simulink model "d3_model_MutiRateAndFractional"  (R2020a)
settings: Solver=VariableStepAuto  StartTime=0.0  StopTime=5e-2  RelTol=1e-3
libraries: dspsigops x6, simulink x2, dspfdesign x1, dspsrcs4 x1
settings Model: Creator=Marat  LastModifiedBy=Marat

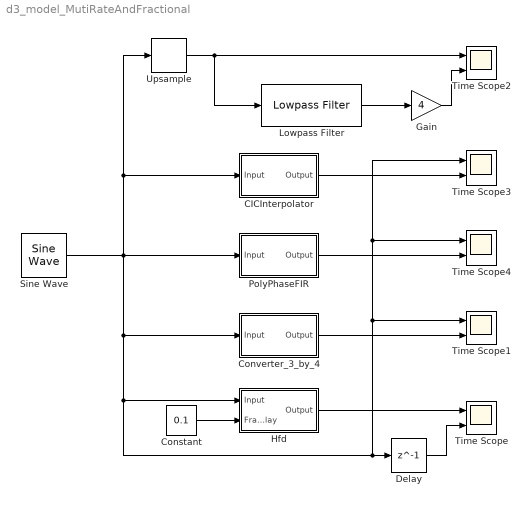
== system d3_model_MutiRateAndFractional ==
  CICInterpolator : Subsystem  Tag=FilterWizardSubSystem
      settings: ErrorFcn=dspFilterRealizedInBasicElemsAlgLoopErrFcnCallback
  Constant : Constant  Value=0.1
  Converter_3_by_4 : Subsystem  Tag=FilterWizardSubSystem
      settings: ErrorFcn=dspFilterRealizedInBasicElemsAlgLoopErrFcnCallback
  Delay : Delay  DelayLength=1
  Gain : Gain  Gain=4
  Hfd : Subsystem  Tag=FilterWizardSubSystem
      settings: ErrorFcn=dspFilterRealizedInBasicElemsAlgLoopErrFcnCallback
  Lowpass Filter : dspfdesign/Lowpass Filter  FilterType=FIR  DesignForMinimumOrder=on  FilterOrder=50  PassbandFrequency=100  StopbandFrequency=500  PassbandRipple=0.1  StopbandAttenuation=40  InheritSampleRate=on  SampleRate=44100  SimulateUsing=Interpreted execution  roundingMode=Floor  coeffsDataTypeStr=fixdt(1,16)
  PolyPhaseFIR : Subsystem  Tag=FilterWizardSubSystem
      settings: ErrorFcn=dspFilterRealizedInBasicElemsAlgLoopErrFcnCallback
  Sine Wave : dspsrcs4/Sine Wave  Amplitude=1  Frequency=50  Phase=0  SampleMode=Discrete  OutComplex=Real  CompMethod=Trigonometric fcn  TableSize=Speed  SampleTime=1/1000  SamplesPerFrame=1  ResetState=Restart at time zero  OutputFrames=off  dataType=double  wordLen=16  udDataType=sfix(16)  fracBitsMode=Best precision  numFracBits=15  OutDataTypeStr=double  LastOutDataTypeStr=double
  Time Scope{,1..4} (5 alike) : Scope  NumInputPorts=2
  Upsample : dspsigops/Upsample  N=4  phase=0  RateOptions=Allow multirate processing  ic=0  mode=Unused parameter value
  wires:
  Sine Wave/1 -> CICInterpolator/1(Input), Upsample/1, Converter_3_by_4/1(Input), Time Scope3/1, Time Scope4/1, Time Scope1/1, Delay/1, Hfd/1(Input), PolyPhaseFIR/1(Input)
  Constant/1 -> Hfd/2(FracDelay)
  Delay/1 -> Time Scope/2
  Converter_3_by_4/1(Output) -> Time Scope1/2
  Upsample/1 -> Time Scope2/1, Lowpass Filter/1
  Gain/1 -> Time Scope2/2
  Lowpass Filter/1 -> Gain/1
  CICInterpolator/1(Output) -> Time Scope3/2
  PolyPhaseFIR/1(Output) -> Time Scope4/2
  Hfd/1(Output) -> Time Scope/1

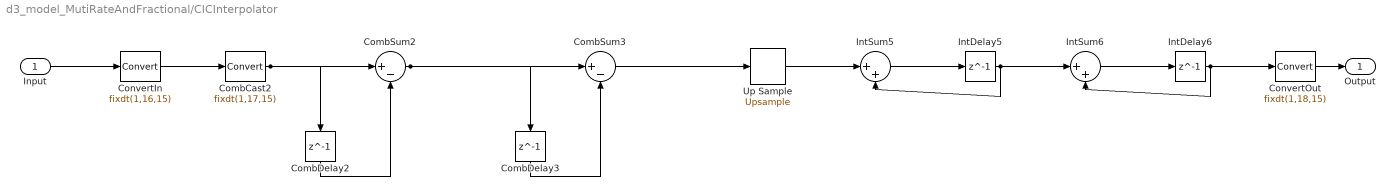
== system d3_model_MutiRateAndFractional/CICInterpolator ==
  Input : Inport
  CombCast2 : DataTypeConversion  OutDataTypeStr=fixdt(1,17,15)
  CombDelay2 : Delay  DelayLength=1  InitialCondition=0
  CombDelay3 : Delay  DelayLength=1  InitialCondition=0
  CombSum2 : Sum  Inputs=|+-  AccumDataTypeStr=fixdt(1,17,15)  OutDataTypeStr=fixdt(1,17,15)
  CombSum3 : Sum  Inputs=|+-  AccumDataTypeStr=fixdt(1,17,15)  OutDataTypeStr=fixdt(1,17,15)
  ConvertIn : DataTypeConversion  OutDataTypeStr=fixdt(1,16,15)  RndMeth=Nearest  SaturateOnIntegerOverflow=on
  ConvertOut : DataTypeConversion  OutDataTypeStr=fixdt(1,18,15)
  IntDelay5 : Delay  DelayLength=1  InitialCondition=0
  IntDelay6 : Delay  DelayLength=1  InitialCondition=0
  IntSum5 : Sum  Inputs=|++  AccumDataTypeStr=fixdt(1,17,15)  OutDataTypeStr=fixdt(1,17,15)
  IntSum6 : Sum  Inputs=|++  AccumDataTypeStr=fixdt(1,18,15)  OutDataTypeStr=fixdt(1,18,15)
  Up Sample : dspsigops/Upsample  N=4  phase=0  RateOptions=Allow multirate processing  ic=0  mode=Unused parameter value
  Output : Outport
  wires:
  Input/1 -> ConvertIn/1
  ConvertIn/1 -> CombCast2/1
  CombSum2/1 -> CombSum3/1, CombDelay3/1
  CombDelay2/1 -> CombSum2/2
  CombCast2/1 -> CombSum2/1, CombDelay2/1
  CombSum3/1 -> Up Sample/1
  CombDelay3/1 -> CombSum3/2
  Up Sample/1 -> IntSum5/1
  IntSum5/1 -> IntDelay5/1
  IntDelay5/1 -> IntSum5/2, IntSum6/1
  IntSum6/1 -> IntDelay6/1
  IntDelay6/1 -> IntSum6/2, ConvertOut/1
  ConvertOut/1 -> Output/1

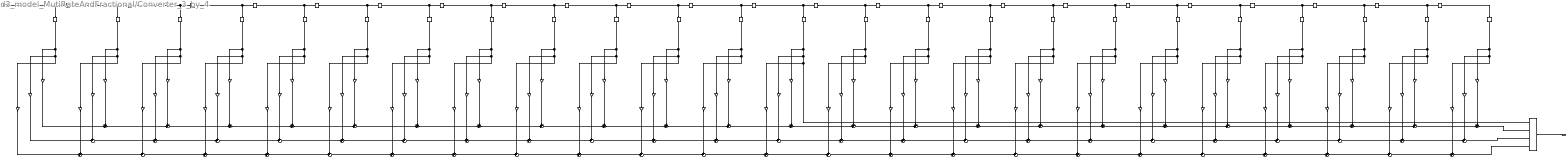
== system d3_model_MutiRateAndFractional/Converter_3_by_4 ==
  Input : Inport
  Delay{2..24} (23 alike) : Delay  DelayLength=1  InitialCondition=0
  FirsrcSys : Subsystem  Tag=FilterWizardSampleRateConverterCommutator
  RT{1..24} (24 alike) : RateTransition  Integrity=off  Deterministic=off  OutPortSampleTimeOpt=Multiple of input port sample time  OutPortSampleTimeMultiple=3/4
  p2(1) : Gain  Gain=-8.94209312709779976e-05  ParamDataTypeStr=double  RndMeth=Nearest  SaturateOnIntegerOverflow=on  OutDataTypeStr=Inherit: Same as input
  p2(10) : Gain  Gain=0.0673410868786561423  ParamDataTypeStr=double  RndMeth=Nearest  SaturateOnIntegerOverflow=on  OutDataTypeStr=Inherit: Same as input
  p2(11) : Gain  Gain=-0.118916504347217039  ParamDataTypeStr=double  RndMeth=Nearest  SaturateOnIntegerOverflow=on  OutDataTypeStr=Inherit: Same as input
  p2(12) : Gain  Gain=0.295831354115615619  ParamDataTypeStr=double  RndMeth=Nearest  SaturateOnIntegerOverflow=on  OutDataTypeStr=Inherit: Same as input
  p2(13) : Gain  Gain=0.898883674956074352  ParamDataTypeStr=double  RndMeth=Nearest  SaturateOnIntegerOverflow=on  OutDataTypeStr=Inherit: Same as input
  p2(14) : Gain  Gain=-0.173018480143057568  ParamDataTypeStr=double  RndMeth=Nearest  SaturateOnIntegerOverflow=on  OutDataTypeStr=Inherit: Same as input
  p2(15) : Gain  Gain=0.0878360099387300586  ParamDataTypeStr=double  RndMeth=Nearest  SaturateOnIntegerOverflow=on  OutDataTypeStr=Inherit: Same as input
  p2(16) : Gain  Gain=-0.0526648923165617677  ParamDataTypeStr=double  RndMeth=Nearest  SaturateOnIntegerOverflow=on  OutDataTypeStr=Inherit: Same as input
  p2(17) : Gain  Gain=0.0329540171313132749  ParamDataTypeStr=double  RndMeth=Nearest  SaturateOnIntegerOverflow=on  OutDataTypeStr=Inherit: Same as input
  p2(18) : Gain  Gain=-0.0205257309215202757  ParamDataTypeStr=double  RndMeth=Nearest  SaturateOnIntegerOverflow=on  OutDataTypeStr=Inherit: Same as input
  p2(19) : Gain  Gain=0.0123854962623023424  ParamDataTypeStr=double  RndMeth=Nearest  SaturateOnIntegerOverflow=on  OutDataTypeStr=Inherit: Same as input
  p2(2) : Gain  Gain=0.000410249281937617467  ParamDataTypeStr=double  RndMeth=Nearest  SaturateOnIntegerOverflow=on  OutDataTypeStr=Inherit: Same as input
  p2(20) : Gain  Gain=-0.00708453163123141071  ParamDataTypeStr=double  RndMeth=Nearest  SaturateOnIntegerOverflow=on  OutDataTypeStr=Inherit: Same as input
  p2(21) : Gain  Gain=0.00375215348431699822  ParamDataTypeStr=double  RndMeth=Nearest  SaturateOnIntegerOverflow=on  OutDataTypeStr=Inherit: Same as input
  p2(22) : Gain  Gain=-0.00178070447416222395  ParamDataTypeStr=double  RndMeth=Nearest  SaturateOnIntegerOverflow=on  OutDataTypeStr=Inherit: Same as input
  p2(23) : Gain  Gain=0.000714756913744617065  ParamDataTypeStr=double  RndMeth=Nearest  SaturateOnIntegerOverflow=on  OutDataTypeStr=Inherit: Same as input
  p2(24) : Gain  Gain=-0.000211174630346201269  ParamDataTypeStr=double  RndMeth=Nearest  SaturateOnIntegerOverflow=on  OutDataTypeStr=Inherit: Same as input
  p2(3) : Gain  Gain=-0.00115837290588860519  ParamDataTypeStr=double  RndMeth=Nearest  SaturateOnIntegerOverflow=on  OutDataTypeStr=Inherit: Same as input
  p2(4) : Gain  Gain=0.00262769403080772646  ParamDataTypeStr=double  RndMeth=Nearest  SaturateOnIntegerOverflow=on  OutDataTypeStr=Inherit: Same as input
  p2(5) : Gain  Gain=-0.00521458482293683193  ParamDataTypeStr=double  RndMeth=Nearest  SaturateOnIntegerOverflow=on  OutDataTypeStr=Inherit: Same as input
  p2(6) : Gain  Gain=0.0094428469685288053  ParamDataTypeStr=double  RndMeth=Nearest  SaturateOnIntegerOverflow=on  OutDataTypeStr=Inherit: Same as input
  p2(7) : Gain  Gain=-0.0160299204416434332  ParamDataTypeStr=double  RndMeth=Nearest  SaturateOnIntegerOverflow=on  OutDataTypeStr=Inherit: Same as input
  p2(8) : Gain  Gain=0.0260729542712553435  ParamDataTypeStr=double  RndMeth=Nearest  SaturateOnIntegerOverflow=on  OutDataTypeStr=Inherit: Same as input
  p2(9) : Gain  Gain=-0.0415922008674667401  ParamDataTypeStr=double  RndMeth=Nearest  SaturateOnIntegerOverflow=on  OutDataTypeStr=Inherit: Same as input
  p3(1) : Gain  Gain=-0.000201076689085048093  ParamDataTypeStr=double  RndMeth=Nearest  SaturateOnIntegerOverflow=on  OutDataTypeStr=Inherit: Same as input
  p3(10) : Gain  Gain=0.108403813182309419  ParamDataTypeStr=double  RndMeth=Nearest  SaturateOnIntegerOverflow=on  OutDataTypeStr=Inherit: Same as input
  p3(11) : Gain  Gain=-0.200342004700688719  ParamDataTypeStr=double  RndMeth=Nearest  SaturateOnIntegerOverflow=on  OutDataTypeStr=Inherit: Same as input
  p3(12) : Gain  Gain=0.632576096651247588  ParamDataTypeStr=double  RndMeth=Nearest  SaturateOnIntegerOverflow=on  OutDataTypeStr=Inherit: Same as input
  p3(13) : Gain  Gain=0.632576096651247588  ParamDataTypeStr=double  RndMeth=Nearest  SaturateOnIntegerOverflow=on  OutDataTypeStr=Inherit: Same as input
  p3(14) : Gain  Gain=-0.200342004700688719  ParamDataTypeStr=double  RndMeth=Nearest  SaturateOnIntegerOverflow=on  OutDataTypeStr=Inherit: Same as input
  p3(15) : Gain  Gain=0.108403813182309419  ParamDataTypeStr=double  RndMeth=Nearest  SaturateOnIntegerOverflow=on  OutDataTypeStr=Inherit: Same as input
  p3(16) : Gain  Gain=-0.0661383425536058861  ParamDataTypeStr=double  RndMeth=Nearest  SaturateOnIntegerOverflow=on  OutDataTypeStr=Inherit: Same as input
  p3(17) : Gain  Gain=0.0414711874768991171  ParamDataTypeStr=double  RndMeth=Nearest  SaturateOnIntegerOverflow=on  OutDataTypeStr=Inherit: Same as input
  p3(18) : Gain  Gain=-0.0256826399041755436  ParamDataTypeStr=double  RndMeth=Nearest  SaturateOnIntegerOverflow=on  OutDataTypeStr=Inherit: Same as input
  p3(19) : Gain  Gain=0.0153221434647724461  ParamDataTypeStr=double  RndMeth=Nearest  SaturateOnIntegerOverflow=on  OutDataTypeStr=Inherit: Same as input
  p3(2) : Gain  Gain=0.000774075413312963327  ParamDataTypeStr=double  RndMeth=Nearest  SaturateOnIntegerOverflow=on  OutDataTypeStr=Inherit: Same as input
  p3(20) : Gain  Gain=-0.00861802747915486021  ParamDataTypeStr=double  RndMeth=Nearest  SaturateOnIntegerOverflow=on  OutDataTypeStr=Inherit: Same as input
  p3(21) : Gain  Gain=0.00445710811660247376  ParamDataTypeStr=double  RndMeth=Nearest  SaturateOnIntegerOverflow=on  OutDataTypeStr=Inherit: Same as input
  p3(22) : Gain  Gain=-0.00204280552852404351  ParamDataTypeStr=double  RndMeth=Nearest  SaturateOnIntegerOverflow=on  OutDataTypeStr=Inherit: Same as input
  p3(23) : Gain  Gain=0.000774075413312963327  ParamDataTypeStr=double  RndMeth=Nearest  SaturateOnIntegerOverflow=on  OutDataTypeStr=Inherit: Same as input
  p3(24) : Gain  Gain=-0.000201076689085048093  ParamDataTypeStr=double  RndMeth=Nearest  SaturateOnIntegerOverflow=on  OutDataTypeStr=Inherit: Same as input
  p3(3) : Gain  Gain=-0.00204280552852404351  ParamDataTypeStr=double  RndMeth=Nearest  SaturateOnIntegerOverflow=on  OutDataTypeStr=Inherit: Same as input
  p3(4) : Gain  Gain=0.00445710811660247376  ParamDataTypeStr=double  RndMeth=Nearest  SaturateOnIntegerOverflow=on  OutDataTypeStr=Inherit: Same as input
  p3(5) : Gain  Gain=-0.00861802747915486021  ParamDataTypeStr=double  RndMeth=Nearest  SaturateOnIntegerOverflow=on  OutDataTypeStr=Inherit: Same as input
  p3(6) : Gain  Gain=0.0153221434647724461  ParamDataTypeStr=double  RndMeth=Nearest  SaturateOnIntegerOverflow=on  OutDataTypeStr=Inherit: Same as input
  p3(7) : Gain  Gain=-0.0256826399041755436  ParamDataTypeStr=double  RndMeth=Nearest  SaturateOnIntegerOverflow=on  OutDataTypeStr=Inherit: Same as input
  p3(8) : Gain  Gain=0.0414711874768991171  ParamDataTypeStr=double  RndMeth=Nearest  SaturateOnIntegerOverflow=on  OutDataTypeStr=Inherit: Same as input
  p3(9) : Gain  Gain=-0.0661383425536058861  ParamDataTypeStr=double  RndMeth=Nearest  SaturateOnIntegerOverflow=on  OutDataTypeStr=Inherit: Same as input
  p4(1) : Gain  Gain=-0.000211174630346201269  ParamDataTypeStr=double  RndMeth=Nearest  SaturateOnIntegerOverflow=on  OutDataTypeStr=Inherit: Same as input
  p4(10) : Gain  Gain=0.0878360099387300586  ParamDataTypeStr=double  RndMeth=Nearest  SaturateOnIntegerOverflow=on  OutDataTypeStr=Inherit: Same as input
  p4(11) : Gain  Gain=-0.173018480143057568  ParamDataTypeStr=double  RndMeth=Nearest  SaturateOnIntegerOverflow=on  OutDataTypeStr=Inherit: Same as input
  p4(12) : Gain  Gain=0.898883674956074352  ParamDataTypeStr=double  RndMeth=Nearest  SaturateOnIntegerOverflow=on  OutDataTypeStr=Inherit: Same as input
  p4(13) : Gain  Gain=0.295831354115615619  ParamDataTypeStr=double  RndMeth=Nearest  SaturateOnIntegerOverflow=on  OutDataTypeStr=Inherit: Same as input
  p4(14) : Gain  Gain=-0.118916504347217039  ParamDataTypeStr=double  RndMeth=Nearest  SaturateOnIntegerOverflow=on  OutDataTypeStr=Inherit: Same as input
  p4(15) : Gain  Gain=0.0673410868786561423  ParamDataTypeStr=double  RndMeth=Nearest  SaturateOnIntegerOverflow=on  OutDataTypeStr=Inherit: Same as input
  p4(16) : Gain  Gain=-0.0415922008674667401  ParamDataTypeStr=double  RndMeth=Nearest  SaturateOnIntegerOverflow=on  OutDataTypeStr=Inherit: Same as input
  p4(17) : Gain  Gain=0.0260729542712553435  ParamDataTypeStr=double  RndMeth=Nearest  SaturateOnIntegerOverflow=on  OutDataTypeStr=Inherit: Same as input
  p4(18) : Gain  Gain=-0.0160299204416434332  ParamDataTypeStr=double  RndMeth=Nearest  SaturateOnIntegerOverflow=on  OutDataTypeStr=Inherit: Same as input
  p4(19) : Gain  Gain=0.0094428469685288053  ParamDataTypeStr=double  RndMeth=Nearest  SaturateOnIntegerOverflow=on  OutDataTypeStr=Inherit: Same as input
  p4(2) : Gain  Gain=0.000714756913744617065  ParamDataTypeStr=double  RndMeth=Nearest  SaturateOnIntegerOverflow=on  OutDataTypeStr=Inherit: Same as input
  p4(20) : Gain  Gain=-0.00521458482293683193  ParamDataTypeStr=double  RndMeth=Nearest  SaturateOnIntegerOverflow=on  OutDataTypeStr=Inherit: Same as input
  p4(21) : Gain  Gain=0.00262769403080772646  ParamDataTypeStr=double  RndMeth=Nearest  SaturateOnIntegerOverflow=on  OutDataTypeStr=Inherit: Same as input
  p4(22) : Gain  Gain=-0.00115837290588860519  ParamDataTypeStr=double  RndMeth=Nearest  SaturateOnIntegerOverflow=on  OutDataTypeStr=Inherit: Same as input
  p4(23) : Gain  Gain=0.000410249281937617467  ParamDataTypeStr=double  RndMeth=Nearest  SaturateOnIntegerOverflow=on  OutDataTypeStr=Inherit: Same as input
  p4(24) : Gain  Gain=-8.94209312709779976e-05  ParamDataTypeStr=double  RndMeth=Nearest  SaturateOnIntegerOverflow=on  OutDataTypeStr=Inherit: Same as input
  p4(3) : Gain  Gain=-0.00178070447416222395  ParamDataTypeStr=double  RndMeth=Nearest  SaturateOnIntegerOverflow=on  OutDataTypeStr=Inherit: Same as input
  p4(4) : Gain  Gain=0.00375215348431699822  ParamDataTypeStr=double  RndMeth=Nearest  SaturateOnIntegerOverflow=on  OutDataTypeStr=Inherit: Same as input
  p4(5) : Gain  Gain=-0.00708453163123141071  ParamDataTypeStr=double  RndMeth=Nearest  SaturateOnIntegerOverflow=on  OutDataTypeStr=Inherit: Same as input
  p4(6) : Gain  Gain=0.0123854962623023424  ParamDataTypeStr=double  RndMeth=Nearest  SaturateOnIntegerOverflow=on  OutDataTypeStr=Inherit: Same as input
  p4(7) : Gain  Gain=-0.0205257309215202757  ParamDataTypeStr=double  RndMeth=Nearest  SaturateOnIntegerOverflow=on  OutDataTypeStr=Inherit: Same as input
  p4(8) : Gain  Gain=0.0329540171313132749  ParamDataTypeStr=double  RndMeth=Nearest  SaturateOnIntegerOverflow=on  OutDataTypeStr=Inherit: Same as input
  p4(9) : Gain  Gain=-0.0526648923165617677  ParamDataTypeStr=double  RndMeth=Nearest  SaturateOnIntegerOverflow=on  OutDataTypeStr=Inherit: Same as input
  sum{62..69,72..79,82..89,610..624,710..724,810..824} (69 alike) : Sum  Inputs=++|  RndMeth=Nearest  SaturateOnIntegerOverflow=on  OutDataTypeStr=Inherit: Same as first input
  Output : Outport
  wires:
  p2(1)/1 -> sum62/2
  p3(1)/1 -> sum72/2
  p4(1)/1 -> sum82/2
  RT1/1 -> p3(1)/1, p4(1)/1, p2(1)/1
  Input/1 -> RT1/1, Delay2/1
  p2(2)/1 -> sum62/1
  p3(2)/1 -> sum72/1
  p4(2)/1 -> sum82/1
  sum62/1 -> sum63/2
  sum72/1 -> sum73/2
  sum82/1 -> sum83/2
  RT2/1 -> p3(2)/1, p4(2)/1, p2(2)/1
  Delay2/1 -> RT2/1, Delay3/1
  p2(3)/1 -> sum63/1
  p3(3)/1 -> sum73/1
  p4(3)/1 -> sum83/1
  sum63/1 -> sum64/2
  sum73/1 -> sum74/2
  sum83/1 -> sum84/2
  RT3/1 -> p3(3)/1, p4(3)/1, p2(3)/1
  Delay3/1 -> RT3/1, Delay4/1
  p2(4)/1 -> sum64/1
  p3(4)/1 -> sum74/1
  p4(4)/1 -> sum84/1
  sum64/1 -> sum65/2
  sum74/1 -> sum75/2
  sum84/1 -> sum85/2
  RT4/1 -> p3(4)/1, p4(4)/1, p2(4)/1
  Delay4/1 -> RT4/1, Delay5/1
  p2(5)/1 -> sum65/1
  p3(5)/1 -> sum75/1
  p4(5)/1 -> sum85/1
  sum65/1 -> sum66/2
  sum75/1 -> sum76/2
  sum85/1 -> sum86/2
  RT5/1 -> p3(5)/1, p4(5)/1, p2(5)/1
  Delay5/1 -> RT5/1, Delay6/1
  p2(6)/1 -> sum66/1
  p3(6)/1 -> sum76/1
  p4(6)/1 -> sum86/1
  sum66/1 -> sum67/2
  sum76/1 -> sum77/2
  sum86/1 -> sum87/2
  RT6/1 -> p3(6)/1, p4(6)/1, p2(6)/1
  Delay6/1 -> RT6/1, Delay7/1
  p2(7)/1 -> sum67/1
  p3(7)/1 -> sum77/1
  p4(7)/1 -> sum87/1
  sum67/1 -> sum68/2
  sum77/1 -> sum78/2
  sum87/1 -> sum88/2
  RT7/1 -> p3(7)/1, p4(7)/1, p2(7)/1
  Delay7/1 -> RT7/1, Delay8/1
  p2(8)/1 -> sum68/1
  p3(8)/1 -> sum78/1
  p4(8)/1 -> sum88/1
  sum68/1 -> sum69/2
  sum78/1 -> sum79/2
  sum88/1 -> sum89/2
  RT8/1 -> p3(8)/1, p4(8)/1, p2(8)/1
  Delay8/1 -> RT8/1, Delay9/1
  p2(9)/1 -> sum69/1
  p3(9)/1 -> sum79/1
  p4(9)/1 -> sum89/1
  sum69/1 -> sum610/2
  sum79/1 -> sum710/2
  sum89/1 -> sum810/2
  RT9/1 -> p3(9)/1, p4(9)/1, p2(9)/1
  Delay9/1 -> RT9/1, Delay10/1
  p2(10)/1 -> sum610/1
  p3(10)/1 -> sum710/1
  p4(10)/1 -> sum810/1
  sum610/1 -> sum611/2
  sum710/1 -> sum711/2
  sum810/1 -> sum811/2
  RT10/1 -> p3(10)/1, p4(10)/1, p2(10)/1
  Delay10/1 -> RT10/1, Delay11/1
  p2(11)/1 -> sum611/1
  p3(11)/1 -> sum711/1
  p4(11)/1 -> sum811/1
  sum611/1 -> sum612/2
  sum711/1 -> sum712/2
  sum811/1 -> sum812/2
  RT11/1 -> p3(11)/1, p4(11)/1, p2(11)/1
  Delay11/1 -> RT11/1, Delay12/1
  p2(12)/1 -> sum612/1
  p3(12)/1 -> sum712/1
  p4(12)/1 -> sum812/1
  sum612/1 -> sum613/2
  sum712/1 -> sum713/2
  sum812/1 -> sum813/2
  RT12/1 -> p3(12)/1, p4(12)/1, p2(12)/1
  Delay12/1 -> RT12/1, Delay13/1
  p2(13)/1 -> sum613/1
  p3(13)/1 -> sum713/1
  p4(13)/1 -> sum813/1
  sum613/1 -> sum614/2
  sum713/1 -> sum714/2
  sum813/1 -> sum814/2
  RT13/1 -> FirsrcSys/1(input1), p4(13)/1, p3(13)/1, p2(13)/1
  Delay13/1 -> RT13/1, Delay14/1
  p2(14)/1 -> sum614/1
  p3(14)/1 -> sum714/1
  p4(14)/1 -> sum814/1
  sum614/1 -> sum615/2
  sum714/1 -> sum715/2
  sum814/1 -> sum815/2
  RT14/1 -> p3(14)/1, p4(14)/1, p2(14)/1
  Delay14/1 -> RT14/1, Delay15/1
  p2(15)/1 -> sum615/1
  p3(15)/1 -> sum715/1
  p4(15)/1 -> sum815/1
  sum615/1 -> sum616/2
  sum715/1 -> sum716/2
  sum815/1 -> sum816/2
  RT15/1 -> p3(15)/1, p4(15)/1, p2(15)/1
  Delay15/1 -> RT15/1, Delay16/1
  p2(16)/1 -> sum616/1
  p3(16)/1 -> sum716/1
  p4(16)/1 -> sum816/1
  sum616/1 -> sum617/2
  sum716/1 -> sum717/2
  sum816/1 -> sum817/2
  RT16/1 -> p3(16)/1, p4(16)/1, p2(16)/1
  Delay16/1 -> RT16/1, Delay17/1
  p2(17)/1 -> sum617/1
  p3(17)/1 -> sum717/1
  p4(17)/1 -> sum817/1
  sum617/1 -> sum618/2
  sum717/1 -> sum718/2
  sum817/1 -> sum818/2
  RT17/1 -> p3(17)/1, p4(17)/1, p2(17)/1
  Delay17/1 -> RT17/1, Delay18/1
  p2(18)/1 -> sum618/1
  p3(18)/1 -> sum718/1
  p4(18)/1 -> sum818/1
  sum618/1 -> sum619/2
  sum718/1 -> sum719/2
  sum818/1 -> sum819/2
  RT18/1 -> p3(18)/1, p4(18)/1, p2(18)/1
  Delay18/1 -> RT18/1, Delay19/1
  p2(19)/1 -> sum619/1
  p3(19)/1 -> sum719/1
  p4(19)/1 -> sum819/1
  sum619/1 -> sum620/2
  sum719/1 -> sum720/2
  sum819/1 -> sum820/2
  RT19/1 -> p3(19)/1, p4(19)/1, p2(19)/1
  Delay19/1 -> RT19/1, Delay20/1
  p2(20)/1 -> sum620/1
  p3(20)/1 -> sum720/1
  p4(20)/1 -> sum820/1
  sum620/1 -> sum621/2
  sum720/1 -> sum721/2
  sum820/1 -> sum821/2
  RT20/1 -> p3(20)/1, p4(20)/1, p2(20)/1
  Delay20/1 -> RT20/1, Delay21/1
  p2(21)/1 -> sum621/1
  p3(21)/1 -> sum721/1
  p4(21)/1 -> sum821/1
  sum621/1 -> sum622/2
  sum721/1 -> sum722/2
  sum821/1 -> sum822/2
  RT21/1 -> p3(21)/1, p4(21)/1, p2(21)/1
  Delay21/1 -> RT21/1, Delay22/1
  p2(22)/1 -> sum622/1
  p3(22)/1 -> sum722/1
  p4(22)/1 -> sum822/1
  sum622/1 -> sum623/2
  sum722/1 -> sum723/2
  sum822/1 -> sum823/2
  RT22/1 -> p3(22)/1, p4(22)/1, p2(22)/1
  Delay22/1 -> RT22/1, Delay23/1
  p2(23)/1 -> sum623/1
  p3(23)/1 -> sum723/1
  p4(23)/1 -> sum823/1
  sum623/1 -> sum624/2
  sum723/1 -> sum724/2
  sum823/1 -> sum824/2
  RT23/1 -> p3(23)/1, p4(23)/1, p2(23)/1
  Delay23/1 -> RT23/1, Delay24/1
  p2(24)/1 -> sum624/1
  p3(24)/1 -> sum724/1
  p4(24)/1 -> sum824/1
  sum624/1 -> FirsrcSys/2(input2)
  sum724/1 -> FirsrcSys/3(input3)
  sum824/1 -> FirsrcSys/4(input4)
  RT24/1 -> p3(24)/1, p4(24)/1, p2(24)/1
  Delay24/1 -> RT24/1
  FirsrcSys/1(output) -> Output/1

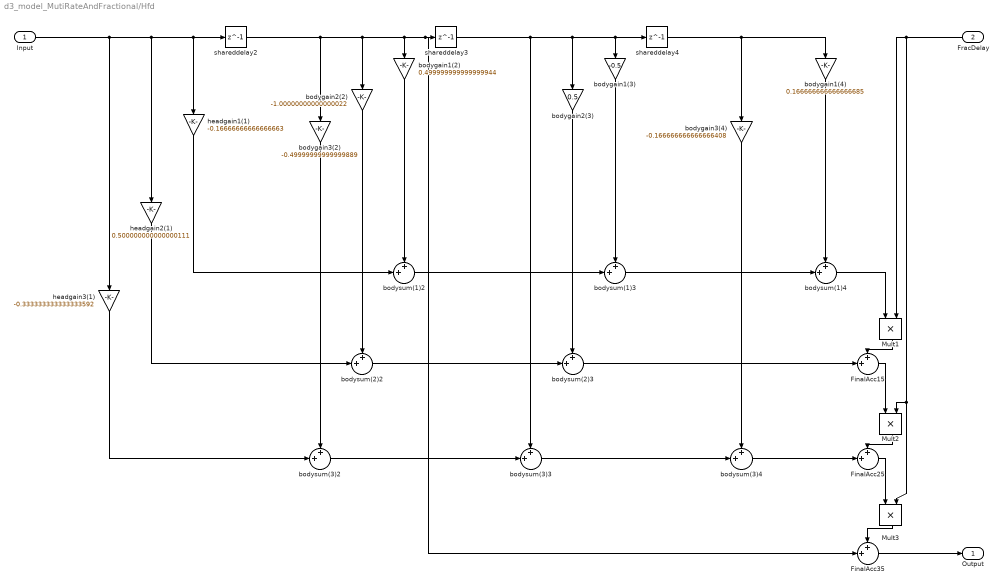
== system d3_model_MutiRateAndFractional/Hfd ==
  Input : Inport
  FracDelay : Inport  Port=2
  FinalAcc15 : Sum  Inputs=++|  RndMeth=Nearest  SaturateOnIntegerOverflow=on  OutDataTypeStr=Inherit: Same as first input
  FinalAcc25 : Sum  Inputs=++|  RndMeth=Nearest  SaturateOnIntegerOverflow=on  OutDataTypeStr=Inherit: Same as first input
  FinalAcc35 : Sum  Inputs=++|  RndMeth=Nearest  SaturateOnIntegerOverflow=on  OutDataTypeStr=Inherit: Same as first input
  Mult1 : Product  RndMeth=Nearest  SaturateOnIntegerOverflow=on  OutDataTypeStr=Inherit: Same as first input
  Mult2 : Product  RndMeth=Nearest  SaturateOnIntegerOverflow=on  OutDataTypeStr=Inherit: Same as first input
  Mult3 : Product  RndMeth=Nearest  SaturateOnIntegerOverflow=on  OutDataTypeStr=Inherit: Same as first input
  bodygain1(2) : Gain  Gain=0.499999999999999944  ParamDataTypeStr=double  RndMeth=Nearest  SaturateOnIntegerOverflow=on  OutDataTypeStr=Inherit: Same as input
  bodygain1(3) : Gain  Gain=-0.5  ParamDataTypeStr=double  RndMeth=Nearest  SaturateOnIntegerOverflow=on  OutDataTypeStr=Inherit: Same as input
  bodygain1(4) : Gain  Gain=0.166666666666666685  ParamDataTypeStr=double  RndMeth=Nearest  SaturateOnIntegerOverflow=on  OutDataTypeStr=Inherit: Same as input
  bodygain2(2) : Gain  Gain=-1.00000000000000022  ParamDataTypeStr=double  RndMeth=Nearest  SaturateOnIntegerOverflow=on  OutDataTypeStr=Inherit: Same as input
  bodygain2(3) : Gain  Gain=0.5  ParamDataTypeStr=double  RndMeth=Nearest  SaturateOnIntegerOverflow=on  OutDataTypeStr=Inherit: Same as input
  bodygain3(2) : Gain  Gain=-0.49999999999999889  ParamDataTypeStr=double  RndMeth=Nearest  SaturateOnIntegerOverflow=on  OutDataTypeStr=Inherit: Same as input
  bodygain3(4) : Gain  Gain=-0.166666666666666408  ParamDataTypeStr=double  RndMeth=Nearest  SaturateOnIntegerOverflow=on  OutDataTypeStr=Inherit: Same as input
  bodysum(1)2 : Sum  Inputs=++|  RndMeth=Nearest  SaturateOnIntegerOverflow=on  OutDataTypeStr=Inherit: Same as first input
  bodysum(1)3 : Sum  Inputs=++|  RndMeth=Nearest  SaturateOnIntegerOverflow=on  OutDataTypeStr=Inherit: Same as first input
  bodysum(1)4 : Sum  Inputs=++|  RndMeth=Nearest  SaturateOnIntegerOverflow=on  OutDataTypeStr=Inherit: Same as first input
  bodysum(2)2 : Sum  Inputs=++|  RndMeth=Nearest  SaturateOnIntegerOverflow=on  OutDataTypeStr=Inherit: Same as first input
  bodysum(2)3 : Sum  Inputs=++|  RndMeth=Nearest  SaturateOnIntegerOverflow=on  OutDataTypeStr=Inherit: Same as first input
  bodysum(3)2 : Sum  Inputs=++|  RndMeth=Nearest  SaturateOnIntegerOverflow=on  OutDataTypeStr=Inherit: Same as first input
  bodysum(3)3 : Sum  Inputs=++|  RndMeth=Nearest  SaturateOnIntegerOverflow=on  OutDataTypeStr=Inherit: Same as first input
  bodysum(3)4 : Sum  Inputs=++|  RndMeth=Nearest  SaturateOnIntegerOverflow=on  OutDataTypeStr=Inherit: Same as first input
  headgain1(1) : Gain  Gain=-0.16666666666666663  ParamDataTypeStr=double  RndMeth=Nearest  SaturateOnIntegerOverflow=on  OutDataTypeStr=Inherit: Same as input
  headgain2(1) : Gain  Gain=0.500000000000000111  ParamDataTypeStr=double  RndMeth=Nearest  SaturateOnIntegerOverflow=on  OutDataTypeStr=Inherit: Same as input
  headgain3(1) : Gain  Gain=-0.333333333333333592  ParamDataTypeStr=double  RndMeth=Nearest  SaturateOnIntegerOverflow=on  OutDataTypeStr=Inherit: Same as input
  shareddelay2 : Delay  DelayLength=1  InitialCondition=0
  shareddelay3 : Delay  DelayLength=1  InitialCondition=0
  shareddelay4 : Delay  DelayLength=1  InitialCondition=0
  Output : Outport
  wires:
  headgain1(1)/1 -> bodysum(1)2/2
  headgain2(1)/1 -> bodysum(2)2/2
  headgain3(1)/1 -> bodysum(3)2/2
  Input/1 -> headgain1(1)/1, shareddelay2/1, headgain2(1)/1, headgain3(1)/1
  bodygain1(2)/1 -> bodysum(1)2/1
  bodygain2(2)/1 -> bodysum(2)2/1
  bodygain3(2)/1 -> bodysum(3)2/1
  bodysum(1)2/1 -> bodysum(1)3/2
  bodysum(2)2/1 -> bodysum(2)3/2
  bodysum(3)2/1 -> bodysum(3)3/2
  shareddelay2/1 -> FinalAcc35/2, shareddelay3/1, bodygain1(2)/1, bodygain2(2)/1, bodygain3(2)/1
  bodygain1(3)/1 -> bodysum(1)3/1
  bodygain2(3)/1 -> bodysum(2)3/1
  bodysum(1)3/1 -> bodysum(1)4/2
  bodysum(2)3/1 -> FinalAcc15/2
  bodysum(3)3/1 -> bodysum(3)4/2
  shareddelay3/1 -> bodygain1(3)/1, shareddelay4/1, bodygain2(3)/1, bodysum(3)3/1
  bodygain1(4)/1 -> bodysum(1)4/1
  bodygain3(4)/1 -> bodysum(3)4/1
  bodysum(1)4/1 -> Mult1/1
  bodysum(3)4/1 -> FinalAcc25/2
  shareddelay4/1 -> bodygain1(4)/1, bodygain3(4)/1
  FracDelay/1 -> Mult2/2, Mult3/2, Mult1/2
  Mult1/1 -> FinalAcc15/1
  FinalAcc15/1 -> Mult2/1
  Mult2/1 -> FinalAcc25/1
  FinalAcc25/1 -> Mult3/1
  Mult3/1 -> FinalAcc35/1
  FinalAcc35/1 -> Output/1

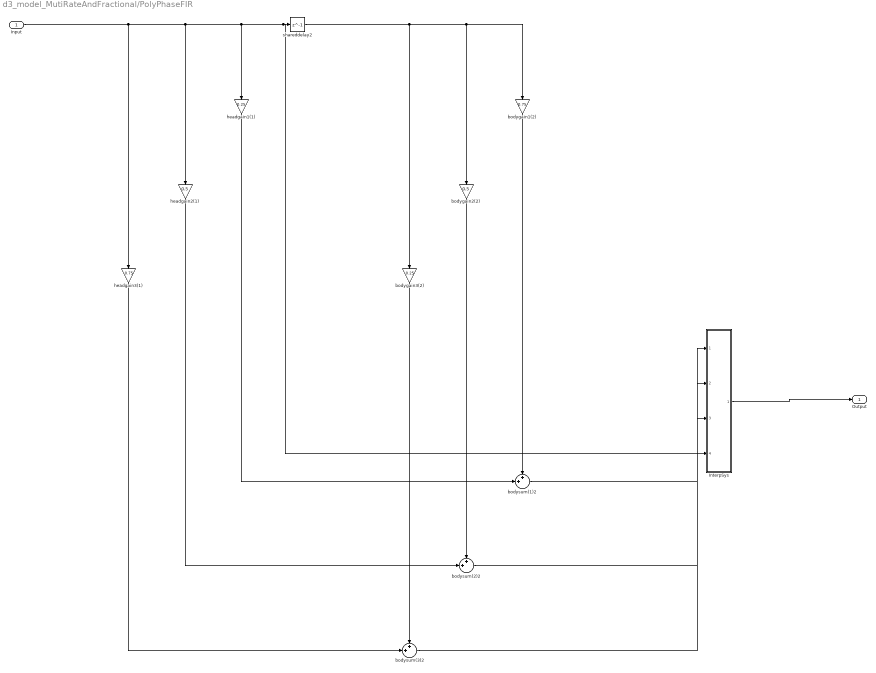
== system d3_model_MutiRateAndFractional/PolyPhaseFIR ==
  Input : Inport
  InterpSys : Subsystem  Tag=FilterWizardInterpolatorCommutator
  bodygain1(2) : Gain  Gain=0.75  ParamDataTypeStr=double  RndMeth=Nearest  SaturateOnIntegerOverflow=on  OutDataTypeStr=Inherit: Same as input
  bodygain2(2) : Gain  Gain=0.5  ParamDataTypeStr=double  RndMeth=Nearest  SaturateOnIntegerOverflow=on  OutDataTypeStr=Inherit: Same as input
  bodygain3(2) : Gain  Gain=0.25  ParamDataTypeStr=double  RndMeth=Nearest  SaturateOnIntegerOverflow=on  OutDataTypeStr=Inherit: Same as input
  bodysum(1)2 : Sum  Inputs=++|  RndMeth=Nearest  SaturateOnIntegerOverflow=on  OutDataTypeStr=Inherit: Same as first input
  bodysum(2)2 : Sum  Inputs=++|  RndMeth=Nearest  SaturateOnIntegerOverflow=on  OutDataTypeStr=Inherit: Same as first input
  bodysum(3)2 : Sum  Inputs=++|  RndMeth=Nearest  SaturateOnIntegerOverflow=on  OutDataTypeStr=Inherit: Same as first input
  headgain1(1) : Gain  Gain=0.25  ParamDataTypeStr=double  RndMeth=Nearest  SaturateOnIntegerOverflow=on  OutDataTypeStr=Inherit: Same as input
  headgain2(1) : Gain  Gain=0.5  ParamDataTypeStr=double  RndMeth=Nearest  SaturateOnIntegerOverflow=on  OutDataTypeStr=Inherit: Same as input
  headgain3(1) : Gain  Gain=0.75  ParamDataTypeStr=double  RndMeth=Nearest  SaturateOnIntegerOverflow=on  OutDataTypeStr=Inherit: Same as input
  shareddelay2 : Delay  DelayLength=1  InitialCondition=0
  Output : Outport
  wires:
  headgain1(1)/1 -> bodysum(1)2/2
  headgain2(1)/1 -> bodysum(2)2/2
  headgain3(1)/1 -> bodysum(3)2/2
  Input/1 -> InterpSys/4(input4), shareddelay2/1, headgain1(1)/1, headgain2(1)/1, headgain3(1)/1
  bodygain1(2)/1 -> bodysum(1)2/1
  bodygain2(2)/1 -> bodysum(2)2/1
  bodygain3(2)/1 -> bodysum(3)2/1
  bodysum(1)2/1 -> InterpSys/1(input1)
  bodysum(2)2/1 -> InterpSys/2(input2)
  bodysum(3)2/1 -> InterpSys/3(input3)
  shareddelay2/1 -> bodygain1(2)/1, bodygain2(2)/1, bodygain3(2)/1
  InterpSys/1(output) -> Output/1

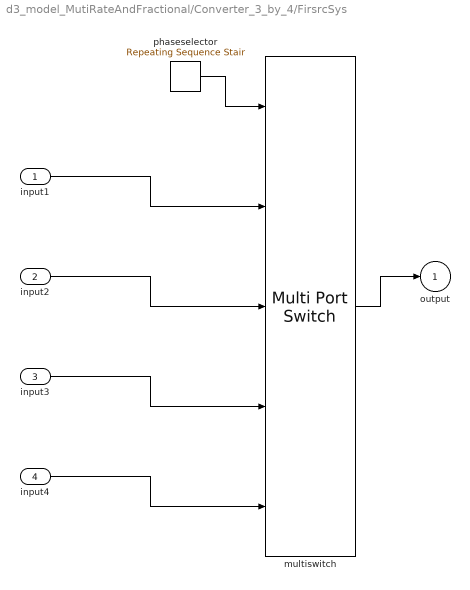
== system d3_model_MutiRateAndFractional/Converter_3_by_4/FirsrcSys ==
  input1 : Inport
  input2 : Inport  Port=2
  input3 : Inport  Port=3
  input4 : Inport  Port=4
  multiswitch : MultiPortSwitch  DataPortOrder=Zero-based contiguous  Inputs=4  zeroidx=on  SaturateOnIntegerOverflow=on
  phaseselector : simulink/Sources/Repeating Sequence Stair  OutValues="[0  3  2  1]"  tsamp=-1  OutMin=[]  OutMax=[]  OutDataTypeStr=double  OutputDataTypeScalingMode=double  OutDataType=fixdt(0,8)  ConRadixGroup=Best Precision: Vector-wise  OutScaling=2^-12
  output : Outport
  wires:
  phaseselector/1 -> multiswitch/1
  input1/1 -> multiswitch/2
  input2/1 -> multiswitch/3
  input3/1 -> multiswitch/4
  input4/1 -> multiswitch/5
  multiswitch/1 -> output/1

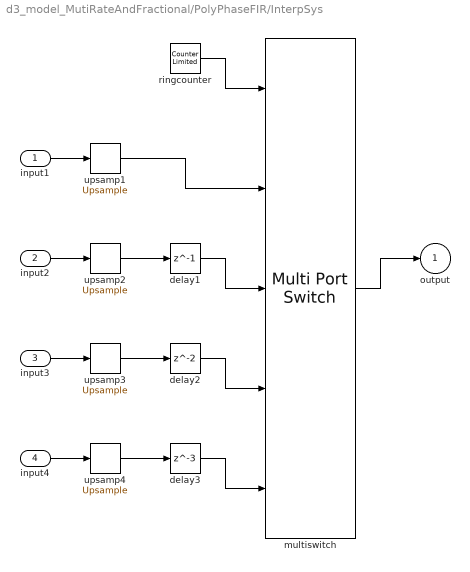
== system d3_model_MutiRateAndFractional/PolyPhaseFIR/InterpSys ==
  input1 : Inport
  input2 : Inport  Port=2
  input3 : Inport  Port=3
  input4 : Inport  Port=4
  delay1 : Delay  DelayLength=1
  delay2 : Delay
  delay3 : Delay  DelayLength=3
  multiswitch : MultiPortSwitch  DataPortOrder=Zero-based contiguous  Inputs=4  zeroidx=on  SaturateOnIntegerOverflow=on
  ringcounter : simulink/Sources/Counter Limited  uplimit=3  tsamp=-1
  upsamp{1..4} (4 alike) : dspsigops/Upsample  N=4  phase=0  RateOptions=Allow multirate processing  ic=0  mode=Unused parameter value
  output : Outport
  wires:
  ringcounter/1 -> multiswitch/1
  input1/1 -> upsamp1/1
  upsamp1/1 -> multiswitch/2
  input2/1 -> upsamp2/1
  upsamp2/1 -> delay1/1
  delay1/1 -> multiswitch/3
  input3/1 -> upsamp3/1
  upsamp3/1 -> delay2/1
  delay2/1 -> multiswitch/4
  input4/1 -> upsamp4/1
  upsamp4/1 -> delay3/1
  delay3/1 -> multiswitch/5
  multiswitch/1 -> output/1
